simulink model "predpreymodel"  (Simulink 7.9)
settings: Solver=ode45  StartTime=0.0  StopTime=10.0  RelTol=1e-6
values from neighbouring files (symbols this model uses):
  a = 2    [predprey.m]
  b = 0.2    [predprey.m]    (also in sir.m = 0.003)
  c = 1    [lim_grow_script.m]    (also in predprey.m = 3)
  d = 0.12    [predprey.m]
  P10 = 80    [predprey.m]
  P20 = 20    [predprey.m]
settings Model: Creator=Daniel  LastModifiedBy=Daniel

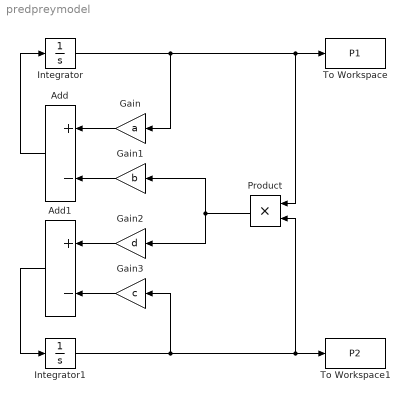
== system predpreymodel ==
  Add : Sum  Inputs=+-
  Add1 : Sum  Inputs=+-
  Gain : Gain  Gain=a
  Gain1 : Gain  Gain=b
  Gain2 : Gain  Gain=d
  Gain3 : Gain  Gain=c
  Integrator : Integrator  InitialCondition=P10
  Integrator1 : Integrator  InitialCondition=P20
  Product : Product  RndMeth=Zero
  To Workspace : ToWorkspace  VariableName=P1  SampleTime=-1
  To Workspace1 : ToWorkspace  VariableName=P2  SampleTime=-1
  wires:
  Add/1 -> Integrator/1
  Add1/1 -> Integrator1/1
  Integrator1/1 -> Gain3/1, Product/2, To Workspace1/1
  Integrator/1 -> Gain/1, Product/1, To Workspace/1
  Gain/1 -> Add/1
  Gain1/1 -> Add/2
  Gain2/1 -> Add1/1
  Gain3/1 -> Add1/2
  Product/1 -> Gain1/1, Gain2/1
